simulink library "ECO_TestLibs"  (R2018a)
settings: Solver=ode45  StartTime=0.0  StopTime=10.0  RelTol=1e-3  EnableMultiTasking=on
undefined symbols (not defined in the file or in its folder): h, km
libraries: CoderSF_BSW_Libs x643, $bdroot x217, SF_CanService_Libs x60, simulink x12
(part 2 of 7)

== system ECO_TestLibs/TAF_CANA/Connected ==
  "Read CAN Message " : SF_CanService_Libs/Read CAN Message  typeCAN=Connected  channel=CAN_A  mEn=off  msgInfo=TAF_CAN_new  msgIterm=CAN0x401x  msgItermStore=CAN0x401x  valid=on  stale=on  motoBit=off  setSignalName=off  defineSignalName=on  prefixSignal='rxCANA'  flgValTest=off  flgNoFixed=off  tSample=Task_L10ms  modeCode=Parameterless
  "Read Fixed-Point CAN Message " : SF_CanService_Libs/Read Fixed-Point CAN Message   typeCAN=Connected  channel=CAN_A  mEn=off  msgInfo=TAF_CAN_new  msgIterm=CAN0x401  msgItermStore=CAN0x401  valid=on  stale=on  motoBit=off  setSignalName=on  defineSignalName=on  prefixSignal='rxCANA'  flgValTest=off  flgNoFixed=off  tSample=Task_L10ms  modeCode=Parameterless
  Subsystem : Subsystem
  Subsystem1 : Subsystem
  Write Measurement1 : CoderSF_BSW_Libs/Calibration & Measurement/Write Measurement  variable_name=TAF_CANF_cntCANARx  variable_value=0  variable_type=uint32  numD=1  unitStr=""  descStr=""
      settings: AttributesFormatString=value:%<variable_value> type:%<variable_type>  SourceProductName=EcoCoder Blocks
  Write Measurement2 : CoderSF_BSW_Libs/Calibration & Measurement/Write Measurement  variable_name=TAF_CAN_cntCANARx  variable_value=0  variable_type=uint32  numD=1  unitStr=""  descStr=""
      settings: AttributesFormatString=value:%<variable_value> type:%<variable_type>  SourceProductName=EcoCoder Blocks
  wires:
  "Read CAN Message "/1 -> Subsystem1/Enable
  "Read CAN Message "/2 -> Write Measurement2/1
  "Read CAN Message "/3 -> Subsystem1/1(In1)
  "Read CAN Message "/4 -> Subsystem1/2(In2)
  "Read CAN Message "/5 -> Subsystem1/3(In3)
  "Read CAN Message "/6 -> Subsystem1/4(In4)
  "Read CAN Message "/7 -> Subsystem1/5(In5)
  "Read CAN Message "/8 -> Subsystem1/6(In6)
  "Read CAN Message "/9 -> Subsystem1/7(In7)
  "Read CAN Message "/10 -> Subsystem1/8(In8)
  "Read Fixed-Point CAN Message "/10 -> Subsystem/8(In8)  "rxCANAByte0"
  "Read Fixed-Point CAN Message "/9 -> Subsystem/7(In7)  "rxCANAByte1"
  "Read Fixed-Point CAN Message "/8 -> Subsystem/6(In6)  "rxCANAByte2"
  "Read Fixed-Point CAN Message "/7 -> Subsystem/5(In5)  "rxCANAByte3"
  "Read Fixed-Point CAN Message "/6 -> Subsystem/4(In4)  "rxCANAByte4"
  "Read Fixed-Point CAN Message "/5 -> Subsystem/3(In3)  "rxCANAByte5"
  "Read Fixed-Point CAN Message "/4 -> Subsystem/2(In2)  "rxCANAByte6"
  "Read Fixed-Point CAN Message "/3 -> Subsystem/1(In1)  "rxCANAByte7"
  "Read Fixed-Point CAN Message "/2 -> Write Measurement1/1
  "Read Fixed-Point CAN Message "/1 -> Subsystem/Enable

== system ECO_TestLibs/TAF_CANA/Disconnected ==
  "Read CAN Message " : SF_CanService_Libs/Read CAN Message  typeCAN=Disconnected  channel=CAN_A  mEn=off  msgInfo=TAF_CAN_new  msgIterm=CAN0x402x  msgItermStore=CAN0x402x  valid=on  stale=on  motoBit=off  setSignalName=off  defineSignalName=on  prefixSignal='rxCANA'  flgValTest=off  flgNoFixed=off  tSample=Task_L10ms  modeCode=Parameterless
  "Read Fixed-Point CAN Message " : SF_CanService_Libs/Read Fixed-Point CAN Message   typeCAN=Disconnected  channel=CAN_A  mEn=off  msgInfo=TAF_CAN_new  msgIterm=CAN0x402  msgItermStore=CAN0x402  valid=on  stale=on  motoBit=off  setSignalName=on  defineSignalName=on  prefixSignal='rxCANA2'  flgValTest=off  flgNoFixed=off  tSample=Task_L10ms  modeCode=Parameterless
  Receive CAN Message : CoderSF_BSW_Libs/CAN/Receive CAN Message  channel=CAN_A  txid=hex2dec('402')  extended=off  txlen=8  tasktimeIndex=Task_Inherit
      settings: SourceProductName=EcoCoder Blocks
  Receive CAN Message1 : CoderSF_BSW_Libs/CAN/Receive CAN Message  channel=CAN_A  txid=hex2dec('412')  extended=on  txlen=8  tasktimeIndex=Task_Inherit
      settings: SourceProductName=EcoCoder Blocks
  Subsystem : Subsystem
  Subsystem1 : Subsystem
  Write Measurement1 : CoderSF_BSW_Libs/Calibration & Measurement/Write Measurement  variable_name=TAF_CANF_cntCANARx2  variable_value=0  variable_type=uint32  numD=1  unitStr=""  descStr=""
      settings: AttributesFormatString=value:%<variable_value> type:%<variable_type>  SourceProductName=EcoCoder Blocks
  Write Measurement2 : CoderSF_BSW_Libs/Calibration & Measurement/Write Measurement  variable_name=TAF_CAN_cntCANARx2  variable_value=0  variable_type=uint32  numD=1  unitStr=""  descStr=""
      settings: AttributesFormatString=value:%<variable_value> type:%<variable_type>  SourceProductName=EcoCoder Blocks
  wires:
  "Read Fixed-Point CAN Message "/1 -> Subsystem/Enable
  "Read Fixed-Point CAN Message "/2 -> Write Measurement1/1
  "Read Fixed-Point CAN Message "/3 -> Subsystem/1(In1)  "rxCANA2Byte7"
  "Read Fixed-Point CAN Message "/4 -> Subsystem/2(In2)  "rxCANA2Byte6"
  "Read Fixed-Point CAN Message "/5 -> Subsystem/3(In3)  "rxCANA2Byte5"
  "Read Fixed-Point CAN Message "/6 -> Subsystem/4(In4)  "rxCANA2Byte4"
  "Read Fixed-Point CAN Message "/7 -> Subsystem/5(In5)  "rxCANA2Byte3"
  "Read Fixed-Point CAN Message "/8 -> Subsystem/6(In6)  "rxCANA2Byte2"
  "Read Fixed-Point CAN Message "/9 -> Subsystem/7(In7)  "rxCANA2Byte1"
  "Read Fixed-Point CAN Message "/10 -> Subsystem/8(In8)  "rxCANA2Byte0"
  "Read CAN Message "/10 -> Subsystem1/8(In8)
  "Read CAN Message "/9 -> Subsystem1/7(In7)
  "Read CAN Message "/8 -> Subsystem1/6(In6)
  "Read CAN Message "/7 -> Subsystem1/5(In5)
  "Read CAN Message "/6 -> Subsystem1/4(In4)
  "Read CAN Message "/5 -> Subsystem1/3(In3)
  "Read CAN Message "/4 -> Subsystem1/2(In2)
  "Read CAN Message "/3 -> Subsystem1/1(In1)
  "Read CAN Message "/2 -> Write Measurement2/1
  "Read CAN Message "/1 -> Subsystem1/Enable
  Receive CAN Message/3 -> "Read Fixed-Point CAN Message "/3
  Receive CAN Message/6 -> "Read Fixed-Point CAN Message "/6
  Receive CAN Message/1 -> "Read Fixed-Point CAN Message "/1
  Receive CAN Message/4 -> "Read Fixed-Point CAN Message "/4
  Receive CAN Message/5 -> "Read Fixed-Point CAN Message "/5
  Receive CAN Message/2 -> "Read Fixed-Point CAN Message "/2
  Receive CAN Message1/3 -> "Read CAN Message "/3
  Receive CAN Message1/4 -> "Read CAN Message "/4
  Receive CAN Message1/2 -> "Read CAN Message "/2
  Receive CAN Message1/5 -> "Read CAN Message "/5
  Receive CAN Message1/1 -> "Read CAN Message "/1
  Receive CAN Message1/6 -> "Read CAN Message "/6

== system ECO_TestLibs/TAF_CANA/Enabled Subsystem ==
  In1 : Inport
  Enable : EnablePort
  "Send CAN Message " : SF_CanService_Libs/Send CAN Message   typeCAN=Connected  channel=CAN_A  mEn=off  msgInfo=TAF_CAN_new  msgIterm=CAN0x7ff  msgItermStore=CAN0x7ff  motoBit=off  flgNoFixed=off  tSample=Task_MDef  modeCode=Parameterless
  Send CAN Message 1 : SF_CanService_Libs/Send CAN Message   typeCAN=Connected  channel=CAN_A  mEn=off  msgInfo=TAF_CAN_new  msgIterm=CAN0x1fffffff  msgItermStore=CAN0x1fffffff  motoBit=off  flgNoFixed=off  tSample=Task_MDef  modeCode=Parameterless
  wires:
  In1/1 -> Send CAN Message 1/1, "Send CAN Message "/1

== system ECO_TestLibs/TAF_CANA/Receive CAN Message ==
  Receive CAN Message : CoderSF_BSW_Libs/CAN/Receive CAN Message  channel=CAN_A  txid=hex2dec('100')  extended=off  txlen=8  tasktimeIndex=Task_L1ms
      settings: SourceProductName=EcoCoder Blocks
  Receive CAN Message1 : CoderSF_BSW_Libs/CAN/Receive CAN Message  channel=CAN_A  txid=hex2dec('100')  extended=off  txlen=8  tasktimeIndex=Task_L1ms
      settings: SourceProductName=EcoCoder Blocks
  Receive CAN Message2 : CoderSF_BSW_Libs/CAN/Receive CAN Message  channel=CAN_A  txid=hex2dec('100')  extended=off  txlen=8  tasktimeIndex=Task_L1ms
      settings: SourceProductName=EcoCoder Blocks
  Write Measurement1 : CoderSF_BSW_Libs/Calibration & Measurement/Write Measurement  variable_name=CANAR1_flgAvailable  variable_value=0  variable_type=boolean  numD=1  unitStr=""  descStr=""
      settings: AttributesFormatString=type:%<variable_type> Dimensions:%<numD>  SourceProductName=EcoCoder Blocks
  Write Measurement10 : CoderSF_BSW_Libs/Calibration & Measurement/Write Measurement  variable_name=CANAR2_id  variable_value=0  variable_type=uint32  numD=1  unitStr=""  descStr=""
      settings: AttributesFormatString=type:%<variable_type> Dimensions:%<numD>  SourceProductName=EcoCoder Blocks
  Write Measurement11 : CoderSF_BSW_Libs/Calibration & Measurement/Write Measurement  variable_name=CANAR2_len  variable_value=0  variable_type=uint8  numD=1  unitStr=""  descStr=""
      settings: AttributesFormatString=type:%<variable_type> Dimensions:%<numD>  SourceProductName=EcoCoder Blocks
  Write Measurement12 : CoderSF_BSW_Libs/Calibration & Measurement/Write Measurement  variable_name=CANAR2_data  variable_value=0  variable_type=uint8  numD=8  unitStr=""  descStr=""
      settings: AttributesFormatString=type:%<variable_type> Dimensions:%<numD>  SourceProductName=EcoCoder Blocks
  Write Measurement13 : CoderSF_BSW_Libs/Calibration & Measurement/Write Measurement  variable_name=CANAR3_id  variable_value=0  variable_type=uint32  numD=1  unitStr=""  descStr=""
      settings: AttributesFormatString=type:%<variable_type> Dimensions:%<numD>  SourceProductName=EcoCoder Blocks
  Write Measurement14 : CoderSF_BSW_Libs/Calibration & Measurement/Write Measurement  variable_name=CANAR3_len  variable_value=0  variable_type=uint8  numD=1  unitStr=""  descStr=""
      settings: AttributesFormatString=type:%<variable_type> Dimensions:%<numD>  SourceProductName=EcoCoder Blocks
  Write Measurement15 : CoderSF_BSW_Libs/Calibration & Measurement/Write Measurement  variable_name=CANAR3_data  variable_value=0  variable_type=uint8  numD=8  unitStr=""  descStr=""
      settings: AttributesFormatString=type:%<variable_type> Dimensions:%<numD>  SourceProductName=EcoCoder Blocks
  Write Measurement16 : CoderSF_BSW_Libs/Calibration & Measurement/Write Measurement  variable_name=CANAR3_flgAvailable  variable_value=0  variable_type=boolean  numD=1  unitStr=""  descStr=""
      settings: AttributesFormatString=type:%<variable_type> Dimensions:%<numD>  SourceProductName=EcoCoder Blocks
  Write Measurement17 : CoderSF_BSW_Libs/Calibration & Measurement/Write Measurement  variable_name=CANAR3_flgRemote  variable_value=0  variable_type=boolean  numD=1  unitStr=""  descStr=""
      settings: AttributesFormatString=type:%<variable_type> Dimensions:%<numD>  SourceProductName=EcoCoder Blocks
  Write Measurement18 : CoderSF_BSW_Libs/Calibration & Measurement/Write Measurement  variable_name=CANAR3_flgExtend  variable_value=0  variable_type=boolean  numD=1  unitStr=""  descStr=""
      settings: AttributesFormatString=type:%<variable_type> Dimensions:%<numD>  SourceProductName=EcoCoder Blocks
  Write Measurement19 : CoderSF_BSW_Libs/Calibration & Measurement/Write Measurement  variable_name=CANAR2_flgExtend  variable_value=0  variable_type=boolean  numD=1  unitStr=""  descStr=""
      settings: AttributesFormatString=type:%<variable_type> Dimensions:%<numD>  SourceProductName=EcoCoder Blocks
  Write Measurement3 : CoderSF_BSW_Libs/Calibration & Measurement/Write Measurement  variable_name=CANAR1_flgRemote  variable_value=0  variable_type=boolean  numD=1  unitStr=""  descStr=""
      settings: AttributesFormatString=type:%<variable_type> Dimensions:%<numD>  SourceProductName=EcoCoder Blocks
  Write Measurement4 : CoderSF_BSW_Libs/Calibration & Measurement/Write Measurement  variable_name=CANAR1_flgExtend  variable_value=0  variable_type=boolean  numD=1  unitStr=""  descStr=""
      settings: AttributesFormatString=type:%<variable_type> Dimensions:%<numD>  SourceProductName=EcoCoder Blocks
  Write Measurement5 : CoderSF_BSW_Libs/Calibration & Measurement/Write Measurement  variable_name=CANAR1_id  variable_value=0  variable_type=uint32  numD=1  unitStr=""  descStr=""
      settings: AttributesFormatString=type:%<variable_type> Dimensions:%<numD>  SourceProductName=EcoCoder Blocks
  Write Measurement6 : CoderSF_BSW_Libs/Calibration & Measurement/Write Measurement  variable_name=CANAR1_len  variable_value=0  variable_type=uint8  numD=1  unitStr=""  descStr=""
      settings: AttributesFormatString=type:%<variable_type> Dimensions:%<numD>  SourceProductName=EcoCoder Blocks
  Write Measurement7 : CoderSF_BSW_Libs/Calibration & Measurement/Write Measurement  variable_name=CANAR1_data  variable_value=0  variable_type=uint8  numD=8  unitStr=""  descStr=""
      settings: AttributesFormatString=type:%<variable_type> Dimensions:%<numD>  SourceProductName=EcoCoder Blocks
  Write Measurement8 : CoderSF_BSW_Libs/Calibration & Measurement/Write Measurement  variable_name=CANAR2_flgAvailable  variable_value=0  variable_type=boolean  numD=1  unitStr=""  descStr=""
      settings: AttributesFormatString=type:%<variable_type> Dimensions:%<numD>  SourceProductName=EcoCoder Blocks
  Write Measurement9 : CoderSF_BSW_Libs/Calibration & Measurement/Write Measurement  variable_name=CANAR2_flgRemote  variable_value=0  variable_type=boolean  numD=1  unitStr=""  descStr=""
      settings: AttributesFormatString=type:%<variable_type> Dimensions:%<numD>  SourceProductName=EcoCoder Blocks
  wires:
  Receive CAN Message/1 -> Write Measurement1/1
  Receive CAN Message/2 -> Write Measurement3/1
  Receive CAN Message/3 -> Write Measurement4/1
  Receive CAN Message/4 -> Write Measurement5/1
  Receive CAN Message/5 -> Write Measurement6/1
  Receive CAN Message/6 -> Write Measurement7/1
  Receive CAN Message1/6 -> Write Measurement12/1
  Receive CAN Message1/4 -> Write Measurement10/1
  Receive CAN Message1/1 -> Write Measurement8/1
  Receive CAN Message1/5 -> Write Measurement11/1
  Receive CAN Message1/2 -> Write Measurement9/1
  Receive CAN Message1/3 -> Write Measurement19/1
  Receive CAN Message2/6 -> Write Measurement15/1
  Receive CAN Message2/4 -> Write Measurement13/1
  Receive CAN Message2/1 -> Write Measurement16/1
  Receive CAN Message2/5 -> Write Measurement14/1
  Receive CAN Message2/2 -> Write Measurement17/1
  Receive CAN Message2/3 -> Write Measurement18/1

== system ECO_TestLibs/TAF_CANA/Subsystem ==
  In1 : Inport
  Logical Operator : Logic  AllPortsSameDT=off  OutDataTypeStr=boolean
  Read Calibration : CoderSF_BSW_Libs/Calibration & Measurement/Read Calibration  variable_name=TAF_CANA_flgEnRxResp_val  variable_value=1  variable_type=boolean  variable_min=[]  variable_max=[]  unitStr=""  descStr=""
      settings: AttributesFormatString=value:%<variable_value> type:%<variable_type> max:%<variable_max> Min:%<variable_min>  SourceProductName=EcoCoder Blocks
  Out1 : Outport
  wires:
  Logical Operator/1 -> Out1/1
  Read Calibration/1 -> Logical Operator/1
  In1/1 -> Logical Operator/2

== system ECO_TestLibs/TAF_CANB/Connected ==
  Read CAN Message 1 : SF_CanService_Libs/Read CAN Message  typeCAN=Connected  channel=CAN_B  mEn=off  msgInfo=TAF_CAN_new  msgIterm=CAN0x403x  msgItermStore=CAN0x403x  valid=on  stale=on  motoBit=off  setSignalName=off  defineSignalName=on  prefixSignal='rxCANB'  flgValTest=off  flgNoFixed=off  tSample=Task_L10ms  modeCode=Parameterless
  Read Fixed-Point CAN Message 1 : SF_CanService_Libs/Read Fixed-Point CAN Message   typeCAN=Connected  channel=CAN_B  mEn=off  msgInfo=TAF_CAN_new  msgIterm=CAN0x403  msgItermStore=CAN0x403  valid=on  stale=on  motoBit=off  setSignalName=on  defineSignalName=on  prefixSignal='rxCANB'  flgValTest=off  flgNoFixed=off  tSample=Task_L10ms  modeCode=Parameterless
  Subsystem1 : Subsystem
  Subsystem5 : Subsystem
  Write Measurement5 : CoderSF_BSW_Libs/Calibration & Measurement/Write Measurement  variable_name=TAF_CAN_cntCANBRx  variable_value=0  variable_type=uint32  numD=1  unitStr=""  descStr=""
      settings: AttributesFormatString=value:%<variable_value> type:%<variable_type>  SourceProductName=EcoCoder Blocks
  Write Measurement6 : CoderSF_BSW_Libs/Calibration & Measurement/Write Measurement  variable_name=TAF_CANF_cntCANBRx  variable_value=0  variable_type=uint32  numD=1  unitStr=""  descStr=""
      settings: AttributesFormatString=value:%<variable_value> type:%<variable_type>  SourceProductName=EcoCoder Blocks
  wires:
  Read Fixed-Point CAN Message 1/4 -> Subsystem1/2(In2)  "rxCANBByte6"
  Read CAN Message 1/1 -> Subsystem5/Enable
  Read CAN Message 1/2 -> Write Measurement5/1
  Read CAN Message 1/3 -> Subsystem5/1(In1)
  Read CAN Message 1/4 -> Subsystem5/2(In2)
  Read CAN Message 1/5 -> Subsystem5/3(In3)
  Read CAN Message 1/6 -> Subsystem5/4(In4)
  Read CAN Message 1/7 -> Subsystem5/5(In5)
  Read CAN Message 1/8 -> Subsystem5/6(In6)
  Read CAN Message 1/9 -> Subsystem5/7(In7)
  Read CAN Message 1/10 -> Subsystem5/8(In8)
  Read Fixed-Point CAN Message 1/10 -> Subsystem1/8(In8)  "rxCANBByte0"
  Read Fixed-Point CAN Message 1/9 -> Subsystem1/7(In7)  "rxCANBByte1"
  Read Fixed-Point CAN Message 1/8 -> Subsystem1/6(In6)  "rxCANBByte2"
  Read Fixed-Point CAN Message 1/7 -> Subsystem1/5(In5)  "rxCANBByte3"
  Read Fixed-Point CAN Message 1/6 -> Subsystem1/4(In4)  "rxCANBByte4"
  Read Fixed-Point CAN Message 1/5 -> Subsystem1/3(In3)  "rxCANBByte5"
  Read Fixed-Point CAN Message 1/3 -> Subsystem1/1(In1)  "rxCANBByte7"
  Read Fixed-Point CAN Message 1/2 -> Write Measurement6/1
  Read Fixed-Point CAN Message 1/1 -> Subsystem1/Enable

== system ECO_TestLibs/TAF_CANB/Disconnected ==
  Read CAN Message 1 : SF_CanService_Libs/Read CAN Message  typeCAN=Disconnected  channel=CAN_B  mEn=off  msgInfo=TAF_CAN_new  msgIterm=CAN0x404x  msgItermStore=CAN0x404x  valid=on  stale=on  motoBit=off  setSignalName=off  defineSignalName=on  prefixSignal='rxCANB'  flgValTest=off  flgNoFixed=off  tSample=Task_L10ms  modeCode=Parameterless
  Read Fixed-Point CAN Message 1 : SF_CanService_Libs/Read Fixed-Point CAN Message   typeCAN=Disconnected  channel=CAN_B  mEn=off  msgInfo=TAF_CAN_new  msgIterm=CAN0x404  msgItermStore=CAN0x404  valid=on  stale=on  motoBit=off  setSignalName=on  defineSignalName=on  prefixSignal='rxCANB2'  flgValTest=off  flgNoFixed=off  tSample=Task_L10ms  modeCode=Parameterless
  Receive CAN Message : CoderSF_BSW_Libs/CAN/Receive CAN Message  channel=CAN_B  txid=hex2dec('404')  extended=off  txlen=8  tasktimeIndex=Task_Inherit
      settings: SourceProductName=EcoCoder Blocks
  Receive CAN Message1 : CoderSF_BSW_Libs/CAN/Receive CAN Message  channel=CAN_B  txid=hex2dec('414')  extended=on  txlen=8  tasktimeIndex=Task_Inherit
      settings: SourceProductName=EcoCoder Blocks
  Subsystem1 : Subsystem
  Subsystem5 : Subsystem
  Write Measurement5 : CoderSF_BSW_Libs/Calibration & Measurement/Write Measurement  variable_name=TAF_CAN_cntCANBRx2  variable_value=0  variable_type=uint32  numD=1  unitStr=""  descStr=""
      settings: AttributesFormatString=value:%<variable_value> type:%<variable_type>  SourceProductName=EcoCoder Blocks
  Write Measurement6 : CoderSF_BSW_Libs/Calibration & Measurement/Write Measurement  variable_name=TAF_CANF_cntCANBRx2  variable_value=0  variable_type=uint32  numD=1  unitStr=""  descStr=""
      settings: AttributesFormatString=value:%<variable_value> type:%<variable_type>  SourceProductName=EcoCoder Blocks
  wires:
  Read Fixed-Point CAN Message 1/1 -> Subsystem1/Enable
  Read Fixed-Point CAN Message 1/2 -> Write Measurement6/1
  Read Fixed-Point CAN Message 1/3 -> Subsystem1/1(In1)  "rxCANB2Byte7"
  Read Fixed-Point CAN Message 1/5 -> Subsystem1/3(In3)  "rxCANB2Byte5"
  Read Fixed-Point CAN Message 1/6 -> Subsystem1/4(In4)  "rxCANB2Byte4"
  Read Fixed-Point CAN Message 1/7 -> Subsystem1/5(In5)  "rxCANB2Byte3"
  Read Fixed-Point CAN Message 1/8 -> Subsystem1/6(In6)  "rxCANB2Byte2"
  Read Fixed-Point CAN Message 1/9 -> Subsystem1/7(In7)  "rxCANB2Byte1"
  Read Fixed-Point CAN Message 1/10 -> Subsystem1/8(In8)  "rxCANB2Byte0"
  Read CAN Message 1/10 -> Subsystem5/8(In8)
  Read CAN Message 1/9 -> Subsystem5/7(In7)
  Read CAN Message 1/8 -> Subsystem5/6(In6)
  Read CAN Message 1/7 -> Subsystem5/5(In5)
  Read CAN Message 1/6 -> Subsystem5/4(In4)
  Read CAN Message 1/5 -> Subsystem5/3(In3)
  Read CAN Message 1/4 -> Subsystem5/2(In2)
  Read CAN Message 1/3 -> Subsystem5/1(In1)
  Read CAN Message 1/2 -> Write Measurement5/1
  Read CAN Message 1/1 -> Subsystem5/Enable
  Read Fixed-Point CAN Message 1/4 -> Subsystem1/2(In2)  "rxCANB2Byte6"
  Receive CAN Message/5 -> Read Fixed-Point CAN Message 1/5
  Receive CAN Message/6 -> Read Fixed-Point CAN Message 1/6
  Receive CAN Message/3 -> Read Fixed-Point CAN Message 1/3
  Receive CAN Message/2 -> Read Fixed-Point CAN Message 1/2
  Receive CAN Message/4 -> Read Fixed-Point CAN Message 1/4
  Receive CAN Message/1 -> Read Fixed-Point CAN Message 1/1
  Receive CAN Message1/3 -> Read CAN Message 1/3
  Receive CAN Message1/5 -> Read CAN Message 1/5
  Receive CAN Message1/2 -> Read CAN Message 1/2
  Receive CAN Message1/1 -> Read CAN Message 1/1
  Receive CAN Message1/6 -> Read CAN Message 1/6
  Receive CAN Message1/4 -> Read CAN Message 1/4

== system ECO_TestLibs/TAF_CANB/Enabled Subsystem ==
  In1 : Inport
  Enable : EnablePort
  "Send CAN Message " : SF_CanService_Libs/Send CAN Message   typeCAN=Connected  channel=CAN_B  mEn=off  msgInfo=TAF_CAN_new  msgIterm=CAN0x7fe  msgItermStore=CAN0x7fe  motoBit=off  flgNoFixed=off  tSample=Task_MDef  modeCode=Parameterless
  Send CAN Message 1 : SF_CanService_Libs/Send CAN Message   typeCAN=Connected  channel=CAN_B  mEn=off  msgInfo=TAF_CAN_new  msgIterm=CAN0x1ffffffe  msgItermStore=CAN0x1ffffffe  motoBit=off  flgNoFixed=off  tSample=Task_MDef  modeCode=Parameterless
  wires:
  In1/1 -> Send CAN Message 1/1, "Send CAN Message "/1

== system ECO_TestLibs/TAF_CANB/Receive CAN Message ==
  Receive CAN Message : CoderSF_BSW_Libs/CAN/Receive CAN Message  channel=CAN_B  txid=hex2dec('100')  extended=off  txlen=8  tasktimeIndex=Task_L1ms
      settings: SourceProductName=EcoCoder Blocks
  Receive CAN Message1 : CoderSF_BSW_Libs/CAN/Receive CAN Message  channel=CAN_B  txid=hex2dec('100')  extended=off  txlen=8  tasktimeIndex=Task_L1ms
      settings: SourceProductName=EcoCoder Blocks
  Receive CAN Message2 : CoderSF_BSW_Libs/CAN/Receive CAN Message  channel=CAN_B  txid=hex2dec('100')  extended=off  txlen=8  tasktimeIndex=Task_L1ms
      settings: SourceProductName=EcoCoder Blocks
  Write Measurement1 : CoderSF_BSW_Libs/Calibration & Measurement/Write Measurement  variable_name=CANBR1_flgAvailable  variable_value=0  variable_type=boolean  numD=1  unitStr=""  descStr=""
      settings: AttributesFormatString=type:%<variable_type> Dimensions:%<numD>  SourceProductName=EcoCoder Blocks
  Write Measurement10 : CoderSF_BSW_Libs/Calibration & Measurement/Write Measurement  variable_name=CANBR2_id  variable_value=0  variable_type=uint32  numD=1  unitStr=""  descStr=""
      settings: AttributesFormatString=type:%<variable_type> Dimensions:%<numD>  SourceProductName=EcoCoder Blocks
  Write Measurement11 : CoderSF_BSW_Libs/Calibration & Measurement/Write Measurement  variable_name=CANBR2_len  variable_value=0  variable_type=uint8  numD=1  unitStr=""  descStr=""
      settings: AttributesFormatString=type:%<variable_type> Dimensions:%<numD>  SourceProductName=EcoCoder Blocks
  Write Measurement12 : CoderSF_BSW_Libs/Calibration & Measurement/Write Measurement  variable_name=CANBR2_data  variable_value=0  variable_type=uint8  numD=8  unitStr=""  descStr=""
      settings: AttributesFormatString=type:%<variable_type> Dimensions:%<numD>  SourceProductName=EcoCoder Blocks
  Write Measurement13 : CoderSF_BSW_Libs/Calibration & Measurement/Write Measurement  variable_name=CANBR3_id  variable_value=0  variable_type=uint32  numD=1  unitStr=""  descStr=""
      settings: AttributesFormatString=type:%<variable_type> Dimensions:%<numD>  SourceProductName=EcoCoder Blocks
  Write Measurement14 : CoderSF_BSW_Libs/Calibration & Measurement/Write Measurement  variable_name=CANBR3_len  variable_value=0  variable_type=uint8  numD=1  unitStr=""  descStr=""
      settings: AttributesFormatString=type:%<variable_type> Dimensions:%<numD>  SourceProductName=EcoCoder Blocks
  Write Measurement15 : CoderSF_BSW_Libs/Calibration & Measurement/Write Measurement  variable_name=CANBR3_data  variable_value=0  variable_type=uint8  numD=8  unitStr=""  descStr=""
      settings: AttributesFormatString=type:%<variable_type> Dimensions:%<numD>  SourceProductName=EcoCoder Blocks
  Write Measurement16 : CoderSF_BSW_Libs/Calibration & Measurement/Write Measurement  variable_name=CANBR3_flgAvailable  variable_value=0  variable_type=boolean  numD=1  unitStr=""  descStr=""
      settings: AttributesFormatString=type:%<variable_type> Dimensions:%<numD>  SourceProductName=EcoCoder Blocks
  Write Measurement17 : CoderSF_BSW_Libs/Calibration & Measurement/Write Measurement  variable_name=CANBR3_flgRemote  variable_value=0  variable_type=boolean  numD=1  unitStr=""  descStr=""
      settings: AttributesFormatString=type:%<variable_type> Dimensions:%<numD>  SourceProductName=EcoCoder Blocks
  Write Measurement18 : CoderSF_BSW_Libs/Calibration & Measurement/Write Measurement  variable_name=CANBR3_flgExtend  variable_value=0  variable_type=boolean  numD=1  unitStr=""  descStr=""
      settings: AttributesFormatString=type:%<variable_type> Dimensions:%<numD>  SourceProductName=EcoCoder Blocks
  Write Measurement19 : CoderSF_BSW_Libs/Calibration & Measurement/Write Measurement  variable_name=CANBR2_flgExtend  variable_value=0  variable_type=boolean  numD=1  unitStr=""  descStr=""
      settings: AttributesFormatString=type:%<variable_type> Dimensions:%<numD>  SourceProductName=EcoCoder Blocks
  Write Measurement3 : CoderSF_BSW_Libs/Calibration & Measurement/Write Measurement  variable_name=CANBR1_flgRemote  variable_value=0  variable_type=boolean  numD=1  unitStr=""  descStr=""
      settings: AttributesFormatString=type:%<variable_type> Dimensions:%<numD>  SourceProductName=EcoCoder Blocks
  Write Measurement4 : CoderSF_BSW_Libs/Calibration & Measurement/Write Measurement  variable_name=CANBR1_flgExtend  variable_value=0  variable_type=boolean  numD=1  unitStr=""  descStr=""
      settings: AttributesFormatString=type:%<variable_type> Dimensions:%<numD>  SourceProductName=EcoCoder Blocks
  Write Measurement5 : CoderSF_BSW_Libs/Calibration & Measurement/Write Measurement  variable_name=CANBR1_id  variable_value=0  variable_type=uint32  numD=1  unitStr=""  descStr=""
      settings: AttributesFormatString=type:%<variable_type> Dimensions:%<numD>  SourceProductName=EcoCoder Blocks
  Write Measurement6 : CoderSF_BSW_Libs/Calibration & Measurement/Write Measurement  variable_name=CANBR1_len  variable_value=0  variable_type=uint8  numD=1  unitStr=""  descStr=""
      settings: AttributesFormatString=type:%<variable_type> Dimensions:%<numD>  SourceProductName=EcoCoder Blocks
  Write Measurement7 : CoderSF_BSW_Libs/Calibration & Measurement/Write Measurement  variable_name=CANBR1_data  variable_value=0  variable_type=uint8  numD=8  unitStr=""  descStr=""
      settings: AttributesFormatString=type:%<variable_type> Dimensions:%<numD>  SourceProductName=EcoCoder Blocks
  Write Measurement8 : CoderSF_BSW_Libs/Calibration & Measurement/Write Measurement  variable_name=CANBR2_flgAvailable  variable_value=0  variable_type=boolean  numD=1  unitStr=""  descStr=""
      settings: AttributesFormatString=type:%<variable_type> Dimensions:%<numD>  SourceProductName=EcoCoder Blocks
  Write Measurement9 : CoderSF_BSW_Libs/Calibration & Measurement/Write Measurement  variable_name=CANBR2_flgRemote  variable_value=0  variable_type=boolean  numD=1  unitStr=""  descStr=""
      settings: AttributesFormatString=type:%<variable_type> Dimensions:%<numD>  SourceProductName=EcoCoder Blocks
  wires:
  Receive CAN Message/1 -> Write Measurement1/1
  Receive CAN Message/2 -> Write Measurement3/1
  Receive CAN Message/3 -> Write Measurement4/1
  Receive CAN Message/4 -> Write Measurement5/1
  Receive CAN Message/5 -> Write Measurement6/1
  Receive CAN Message/6 -> Write Measurement7/1
  Receive CAN Message1/6 -> Write Measurement12/1
  Receive CAN Message1/4 -> Write Measurement10/1
  Receive CAN Message1/1 -> Write Measurement8/1
  Receive CAN Message1/5 -> Write Measurement11/1
  Receive CAN Message1/2 -> Write Measurement9/1
  Receive CAN Message1/3 -> Write Measurement19/1
  Receive CAN Message2/6 -> Write Measurement15/1
  Receive CAN Message2/4 -> Write Measurement13/1
  Receive CAN Message2/1 -> Write Measurement16/1
  Receive CAN Message2/5 -> Write Measurement14/1
  Receive CAN Message2/2 -> Write Measurement17/1
  Receive CAN Message2/3 -> Write Measurement18/1

== system ECO_TestLibs/TAF_CANB/Subsystem ==
  In1 : Inport
  Logical Operator : Logic  AllPortsSameDT=off  OutDataTypeStr=boolean
  Read Calibration : CoderSF_BSW_Libs/Calibration & Measurement/Read Calibration  variable_name=TAF_CANB_flgEnRxResp_val  variable_value=1  variable_type=boolean  variable_min=[]  variable_max=[]  unitStr=""  descStr=""
      settings: AttributesFormatString=value:%<variable_value> type:%<variable_type> max:%<variable_max> Min:%<variable_min>  SourceProductName=EcoCoder Blocks
  Out1 : Outport
  wires:
  Logical Operator/1 -> Out1/1
  Read Calibration/1 -> Logical Operator/1
  In1/1 -> Logical Operator/2

== system ECO_TestLibs/TAF_CANC/Connected ==
  Read CAN Message 2 : SF_CanService_Libs/Read CAN Message  typeCAN=Connected  channel=CAN_C  mEn=off  msgInfo=TAF_CAN_new  msgIterm=CAN0x405x  msgItermStore=CAN0x405x  valid=on  stale=on  motoBit=off  setSignalName=off  defineSignalName=on  prefixSignal='rxCANC'  flgValTest=off  flgNoFixed=off  tSample=Task_L10ms  modeCode=Parameterless
  Read Fixed-Point CAN Message 2 : SF_CanService_Libs/Read Fixed-Point CAN Message   typeCAN=Connected  channel=CAN_C  mEn=off  msgInfo=TAF_CAN_new  msgIterm=CAN0x405  msgItermStore=CAN0x405  valid=on  stale=on  motoBit=off  setSignalName=on  defineSignalName=on  prefixSignal='rxCANC'  flgValTest=off  flgNoFixed=off  tSample=Task_L10ms  modeCode=Parameterless
  Subsystem2 : Subsystem
  Subsystem6 : Subsystem
  Write Measurement10 : CoderSF_BSW_Libs/Calibration & Measurement/Write Measurement  variable_name=TAF_CAN_cntCANCRx  variable_value=0  variable_type=uint32  numD=1  unitStr=""  descStr=""
      settings: AttributesFormatString=value:%<variable_value> type:%<variable_type>  SourceProductName=EcoCoder Blocks
  Write Measurement7 : CoderSF_BSW_Libs/Calibration & Measurement/Write Measurement  variable_name=TAF_CANF_cntCANCRx  variable_value=0  variable_type=uint32  numD=1  unitStr=""  descStr=""
      settings: AttributesFormatString=value:%<variable_value> type:%<variable_type>  SourceProductName=EcoCoder Blocks
  wires:
  Read Fixed-Point CAN Message 2/1 -> Subsystem2/Enable
  Read Fixed-Point CAN Message 2/2 -> Write Measurement7/1
  Read Fixed-Point CAN Message 2/3 -> Subsystem2/1(In1)  "rxCANCByte7"
  Read Fixed-Point CAN Message 2/4 -> Subsystem2/2(In2)  "rxCANCByte6"
  Read Fixed-Point CAN Message 2/5 -> Subsystem2/3(In3)  "rxCANCByte5"
  Read Fixed-Point CAN Message 2/6 -> Subsystem2/4(In4)  "rxCANCByte4"
  Read Fixed-Point CAN Message 2/7 -> Subsystem2/5(In5)  "rxCANCByte3"
  Read Fixed-Point CAN Message 2/8 -> Subsystem2/6(In6)  "rxCANCByte2"
  Read Fixed-Point CAN Message 2/9 -> Subsystem2/7(In7)  "rxCANCByte1"
  Read Fixed-Point CAN Message 2/10 -> Subsystem2/8(In8)  "rxCANCByte0"
  Read CAN Message 2/10 -> Subsystem6/8(In8)
  Read CAN Message 2/9 -> Subsystem6/7(In7)
  Read CAN Message 2/8 -> Subsystem6/6(In6)
  Read CAN Message 2/7 -> Subsystem6/5(In5)
  Read CAN Message 2/6 -> Subsystem6/4(In4)
  Read CAN Message 2/5 -> Subsystem6/3(In3)
  Read CAN Message 2/4 -> Subsystem6/2(In2)
  Read CAN Message 2/3 -> Subsystem6/1(In1)
  Read CAN Message 2/2 -> Write Measurement10/1
  Read CAN Message 2/1 -> Subsystem6/Enable

== system ECO_TestLibs/TAF_CANC/Disconnected ==
  Read CAN Message 2 : SF_CanService_Libs/Read CAN Message  typeCAN=Disconnected  channel=CAN_C  mEn=off  msgInfo=TAF_CAN_new  msgIterm=CAN0x406x  msgItermStore=CAN0x406x  valid=on  stale=on  motoBit=off  setSignalName=off  defineSignalName=on  prefixSignal='rxCANC'  flgValTest=off  flgNoFixed=off  tSample=Task_L10ms  modeCode=Parameterless
  Read Fixed-Point CAN Message 2 : SF_CanService_Libs/Read Fixed-Point CAN Message   typeCAN=Disconnected  channel=CAN_C  mEn=off  msgInfo=TAF_CAN_new  msgIterm=CAN0x406  msgItermStore=CAN0x406  valid=on  stale=on  motoBit=off  setSignalName=on  defineSignalName=on  prefixSignal='rxCANC2'  flgValTest=off  flgNoFixed=off  tSample=Task_L10ms  modeCode=Parameterless
  Receive CAN Message : CoderSF_BSW_Libs/CAN/Receive CAN Message  channel=CAN_C  txid=hex2dec('406')  extended=off  txlen=8  tasktimeIndex=Task_Inherit
      settings: SourceProductName=EcoCoder Blocks
  Receive CAN Message1 : CoderSF_BSW_Libs/CAN/Receive CAN Message  channel=CAN_C  txid=hex2dec('416')  extended=on  txlen=8  tasktimeIndex=Task_Inherit
      settings: SourceProductName=EcoCoder Blocks
  Subsystem2 : Subsystem
  Subsystem6 : Subsystem
  Write Measurement10 : CoderSF_BSW_Libs/Calibration & Measurement/Write Measurement  variable_name=TAF_CAN_cntCANCRx2  variable_value=0  variable_type=uint32  numD=1  unitStr=""  descStr=""
      settings: AttributesFormatString=value:%<variable_value> type:%<variable_type>  SourceProductName=EcoCoder Blocks
  Write Measurement7 : CoderSF_BSW_Libs/Calibration & Measurement/Write Measurement  variable_name=TAF_CANF_cntCANCRx2  variable_value=0  variable_type=uint32  numD=1  unitStr=""  descStr=""
      settings: AttributesFormatString=value:%<variable_value> type:%<variable_type>  SourceProductName=EcoCoder Blocks
  wires:
  Read CAN Message 2/1 -> Subsystem6/Enable
  Read CAN Message 2/2 -> Write Measurement10/1
  Read CAN Message 2/3 -> Subsystem6/1(In1)
  Read CAN Message 2/4 -> Subsystem6/2(In2)
  Read CAN Message 2/5 -> Subsystem6/3(In3)
  Read CAN Message 2/6 -> Subsystem6/4(In4)
  Read CAN Message 2/7 -> Subsystem6/5(In5)
  Read CAN Message 2/8 -> Subsystem6/6(In6)
  Read CAN Message 2/9 -> Subsystem6/7(In7)
  Read CAN Message 2/10 -> Subsystem6/8(In8)
  Read Fixed-Point CAN Message 2/10 -> Subsystem2/8(In8)  "rxCANC2Byte0"
  Read Fixed-Point CAN Message 2/9 -> Subsystem2/7(In7)  "rxCANC2Byte1"
  Read Fixed-Point CAN Message 2/8 -> Subsystem2/6(In6)  "rxCANC2Byte2"
  Read Fixed-Point CAN Message 2/7 -> Subsystem2/5(In5)  "rxCANC2Byte3"
  Read Fixed-Point CAN Message 2/6 -> Subsystem2/4(In4)  "rxCANC2Byte4"
  Read Fixed-Point CAN Message 2/5 -> Subsystem2/3(In3)  "rxCANC2Byte5"
  Read Fixed-Point CAN Message 2/4 -> Subsystem2/2(In2)  "rxCANC2Byte6"
  Read Fixed-Point CAN Message 2/3 -> Subsystem2/1(In1)  "rxCANC2Byte7"
  Read Fixed-Point CAN Message 2/2 -> Write Measurement7/1
  Read Fixed-Point CAN Message 2/1 -> Subsystem2/Enable
  Receive CAN Message/1 -> Read Fixed-Point CAN Message 2/1
  Receive CAN Message/6 -> Read Fixed-Point CAN Message 2/6
  Receive CAN Message/2 -> Read Fixed-Point CAN Message 2/2
  Receive CAN Message/5 -> Read Fixed-Point CAN Message 2/5
  Receive CAN Message/4 -> Read Fixed-Point CAN Message 2/4
  Receive CAN Message/3 -> Read Fixed-Point CAN Message 2/3
  Receive CAN Message1/1 -> Read CAN Message 2/1
  Receive CAN Message1/4 -> Read CAN Message 2/4
  Receive CAN Message1/5 -> Read CAN Message 2/5
  Receive CAN Message1/6 -> Read CAN Message 2/6
  Receive CAN Message1/3 -> Read CAN Message 2/3
  Receive CAN Message1/2 -> Read CAN Message 2/2

== system ECO_TestLibs/TAF_CANC/Enabled Subsystem ==
  In1 : Inport
  Enable : EnablePort
  "Send CAN Message " : SF_CanService_Libs/Send CAN Message   typeCAN=Connected  channel=CAN_C  mEn=off  msgInfo=TAF_CAN_new  msgIterm=CAN0x7fd  msgItermStore=CAN0x7fd  motoBit=off  flgNoFixed=off  tSample=Task_MDef  modeCode=Parameterless
  Send CAN Message 1 : SF_CanService_Libs/Send CAN Message   typeCAN=Connected  channel=CAN_C  mEn=off  msgInfo=TAF_CAN_new  msgIterm=CAN0x1ffffffd  msgItermStore=CAN0x1ffffffd  motoBit=off  flgNoFixed=off  tSample=Task_MDef  modeCode=Parameterless
  wires:
  In1/1 -> Send CAN Message 1/1, "Send CAN Message "/1

== system ECO_TestLibs/TAF_CANC/Receive CAN Message ==
  Receive CAN Message : CoderSF_BSW_Libs/CAN/Receive CAN Message  channel=CAN_C  txid=hex2dec('100')  extended=off  txlen=8  tasktimeIndex=Task_L1ms
      settings: SourceProductName=EcoCoder Blocks
  Receive CAN Message1 : CoderSF_BSW_Libs/CAN/Receive CAN Message  channel=CAN_C  txid=hex2dec('100')  extended=off  txlen=8  tasktimeIndex=Task_L1ms
      settings: SourceProductName=EcoCoder Blocks
  Receive CAN Message2 : CoderSF_BSW_Libs/CAN/Receive CAN Message  channel=CAN_C  txid=hex2dec('100')  extended=off  txlen=8  tasktimeIndex=Task_L1ms
      settings: SourceProductName=EcoCoder Blocks
  Write Measurement1 : CoderSF_BSW_Libs/Calibration & Measurement/Write Measurement  variable_name=CANCR1_flgAvailable  variable_value=0  variable_type=boolean  numD=1  unitStr=""  descStr=""
      settings: AttributesFormatString=type:%<variable_type> Dimensions:%<numD>  SourceProductName=EcoCoder Blocks
  Write Measurement10 : CoderSF_BSW_Libs/Calibration & Measurement/Write Measurement  variable_name=CANCR2_id  variable_value=0  variable_type=uint32  numD=1  unitStr=""  descStr=""
      settings: AttributesFormatString=type:%<variable_type> Dimensions:%<numD>  SourceProductName=EcoCoder Blocks
  Write Measurement11 : CoderSF_BSW_Libs/Calibration & Measurement/Write Measurement  variable_name=CANCR2_len  variable_value=0  variable_type=uint8  numD=1  unitStr=""  descStr=""
      settings: AttributesFormatString=type:%<variable_type> Dimensions:%<numD>  SourceProductName=EcoCoder Blocks
  Write Measurement12 : CoderSF_BSW_Libs/Calibration & Measurement/Write Measurement  variable_name=CANCR2_data  variable_value=0  variable_type=uint8  numD=8  unitStr=""  descStr=""
      settings: AttributesFormatString=type:%<variable_type> Dimensions:%<numD>  SourceProductName=EcoCoder Blocks
  Write Measurement13 : CoderSF_BSW_Libs/Calibration & Measurement/Write Measurement  variable_name=CANCR3_id  variable_value=0  variable_type=uint32  numD=1  unitStr=""  descStr=""
      settings: AttributesFormatString=type:%<variable_type> Dimensions:%<numD>  SourceProductName=EcoCoder Blocks
  Write Measurement14 : CoderSF_BSW_Libs/Calibration & Measurement/Write Measurement  variable_name=CANCR3_len  variable_value=0  variable_type=uint8  numD=1  unitStr=""  descStr=""
      settings: AttributesFormatString=type:%<variable_type> Dimensions:%<numD>  SourceProductName=EcoCoder Blocks
  Write Measurement15 : CoderSF_BSW_Libs/Calibration & Measurement/Write Measurement  variable_name=CANCR3_data  variable_value=0  variable_type=uint8  numD=8  unitStr=""  descStr=""
      settings: AttributesFormatString=type:%<variable_type> Dimensions:%<numD>  SourceProductName=EcoCoder Blocks
  Write Measurement16 : CoderSF_BSW_Libs/Calibration & Measurement/Write Measurement  variable_name=CANCR3_flgAvailable  variable_value=0  variable_type=boolean  numD=1  unitStr=""  descStr=""
      settings: AttributesFormatString=type:%<variable_type> Dimensions:%<numD>  SourceProductName=EcoCoder Blocks
  Write Measurement17 : CoderSF_BSW_Libs/Calibration & Measurement/Write Measurement  variable_name=CANCR3_flgRemote  variable_value=0  variable_type=boolean  numD=1  unitStr=""  descStr=""
      settings: AttributesFormatString=type:%<variable_type> Dimensions:%<numD>  SourceProductName=EcoCoder Blocks
  Write Measurement18 : CoderSF_BSW_Libs/Calibration & Measurement/Write Measurement  variable_name=CANCR3_flgExtend  variable_value=0  variable_type=boolean  numD=1  unitStr=""  descStr=""
      settings: AttributesFormatString=type:%<variable_type> Dimensions:%<numD>  SourceProductName=EcoCoder Blocks
  Write Measurement19 : CoderSF_BSW_Libs/Calibration & Measurement/Write Measurement  variable_name=CANCR2_flgExtend  variable_value=0  variable_type=boolean  numD=1  unitStr=""  descStr=""
      settings: AttributesFormatString=type:%<variable_type> Dimensions:%<numD>  SourceProductName=EcoCoder Blocks
  Write Measurement3 : CoderSF_BSW_Libs/Calibration & Measurement/Write Measurement  variable_name=CANCR1_flgRemote  variable_value=0  variable_type=boolean  numD=1  unitStr=""  descStr=""
      settings: AttributesFormatString=type:%<variable_type> Dimensions:%<numD>  SourceProductName=EcoCoder Blocks
  Write Measurement4 : CoderSF_BSW_Libs/Calibration & Measurement/Write Measurement  variable_name=CANCR1_flgExtend  variable_value=0  variable_type=boolean  numD=1  unitStr=""  descStr=""
      settings: AttributesFormatString=type:%<variable_type> Dimensions:%<numD>  SourceProductName=EcoCoder Blocks
  Write Measurement5 : CoderSF_BSW_Libs/Calibration & Measurement/Write Measurement  variable_name=CANCR1_id  variable_value=0  variable_type=uint32  numD=1  unitStr=""  descStr=""
      settings: AttributesFormatString=type:%<variable_type> Dimensions:%<numD>  SourceProductName=EcoCoder Blocks
  Write Measurement6 : CoderSF_BSW_Libs/Calibration & Measurement/Write Measurement  variable_name=CANCR1_len  variable_value=0  variable_type=uint8  numD=1  unitStr=""  descStr=""
      settings: AttributesFormatString=type:%<variable_type> Dimensions:%<numD>  SourceProductName=EcoCoder Blocks
  Write Measurement7 : CoderSF_BSW_Libs/Calibration & Measurement/Write Measurement  variable_name=CANCR1_data  variable_value=0  variable_type=uint8  numD=8  unitStr=""  descStr=""
      settings: AttributesFormatString=type:%<variable_type> Dimensions:%<numD>  SourceProductName=EcoCoder Blocks
  Write Measurement8 : CoderSF_BSW_Libs/Calibration & Measurement/Write Measurement  variable_name=CANCR2_flgAvailable  variable_value=0  variable_type=boolean  numD=1  unitStr=""  descStr=""
      settings: AttributesFormatString=type:%<variable_type> Dimensions:%<numD>  SourceProductName=EcoCoder Blocks
  Write Measurement9 : CoderSF_BSW_Libs/Calibration & Measurement/Write Measurement  variable_name=CANCR2_flgRemote  variable_value=0  variable_type=boolean  numD=1  unitStr=""  descStr=""
      settings: AttributesFormatString=type:%<variable_type> Dimensions:%<numD>  SourceProductName=EcoCoder Blocks
  wires:
  Receive CAN Message/1 -> Write Measurement1/1
  Receive CAN Message/2 -> Write Measurement3/1
  Receive CAN Message/3 -> Write Measurement4/1
  Receive CAN Message/4 -> Write Measurement5/1
  Receive CAN Message/5 -> Write Measurement6/1
  Receive CAN Message/6 -> Write Measurement7/1
  Receive CAN Message1/6 -> Write Measurement12/1
  Receive CAN Message1/4 -> Write Measurement10/1
  Receive CAN Message1/1 -> Write Measurement8/1
  Receive CAN Message1/5 -> Write Measurement11/1
  Receive CAN Message1/2 -> Write Measurement9/1
  Receive CAN Message1/3 -> Write Measurement19/1
  Receive CAN Message2/6 -> Write Measurement15/1
  Receive CAN Message2/4 -> Write Measurement13/1
  Receive CAN Message2/1 -> Write Measurement16/1
  Receive CAN Message2/5 -> Write Measurement14/1
  Receive CAN Message2/2 -> Write Measurement17/1
  Receive CAN Message2/3 -> Write Measurement18/1

== system ECO_TestLibs/TAF_CANC/Subsystem ==
  In1 : Inport
  Logical Operator : Logic  AllPortsSameDT=off  OutDataTypeStr=boolean
  Read Calibration : CoderSF_BSW_Libs/Calibration & Measurement/Read Calibration  variable_name=TAF_CANC_flgEnRxResp_val  variable_value=1  variable_type=boolean  variable_min=[]  variable_max=[]  unitStr=""  descStr=""
      settings: AttributesFormatString=value:%<variable_value> type:%<variable_type> max:%<variable_max> Min:%<variable_min>  SourceProductName=EcoCoder Blocks
  Out1 : Outport
  wires:
  Logical Operator/1 -> Out1/1
  Read Calibration/1 -> Logical Operator/1
  In1/1 -> Logical Operator/2

== system ECO_TestLibs/TAF_CAND/Connected ==
  Read CAN Message 3 : SF_CanService_Libs/Read CAN Message  typeCAN=Connected  channel=CAN_D  mEn=off  msgInfo=TAF_CAN_new  msgIterm=CAN0x407x  msgItermStore=CAN0x407x  valid=on  stale=on  motoBit=off  setSignalName=off  defineSignalName=on  prefixSignal='rxCAND'  flgValTest=off  flgNoFixed=off  tSample=Task_L10ms  modeCode=Parameterless
  Read Fixed-Point CAN Message 3 : SF_CanService_Libs/Read Fixed-Point CAN Message   typeCAN=Connected  channel=CAN_D  mEn=off  msgInfo=TAF_CAN_new  msgIterm=CAN0x407  msgItermStore=CAN0x407  valid=on  stale=on  motoBit=off  setSignalName=on  defineSignalName=on  prefixSignal='rxCAND'  flgValTest=off  flgNoFixed=off  tSample=Task_L10ms  modeCode=Parameterless
  Subsystem3 : Subsystem
  Subsystem7 : Subsystem
  Write Measurement11 : CoderSF_BSW_Libs/Calibration & Measurement/Write Measurement  variable_name=TAF_CAN_cntCANDRx  variable_value=0  variable_type=uint32  numD=1  unitStr=""  descStr=""
      settings: AttributesFormatString=value:%<variable_value> type:%<variable_type>  SourceProductName=EcoCoder Blocks
  Write Measurement8 : CoderSF_BSW_Libs/Calibration & Measurement/Write Measurement  variable_name=TAF_CANF_cntCANDRx  variable_value=0  variable_type=uint32  numD=1  unitStr=""  descStr=""
      settings: AttributesFormatString=value:%<variable_value> type:%<variable_type>  SourceProductName=EcoCoder Blocks
  wires:
  Read CAN Message 3/1 -> Subsystem7/Enable
  Read CAN Message 3/2 -> Write Measurement11/1
  Read CAN Message 3/3 -> Subsystem7/1(In1)
  Read CAN Message 3/4 -> Subsystem7/2(In2)
  Read CAN Message 3/5 -> Subsystem7/3(In3)
  Read CAN Message 3/6 -> Subsystem7/4(In4)
  Read CAN Message 3/7 -> Subsystem7/5(In5)
  Read CAN Message 3/8 -> Subsystem7/6(In6)
  Read CAN Message 3/9 -> Subsystem7/7(In7)
  Read CAN Message 3/10 -> Subsystem7/8(In8)
  Read Fixed-Point CAN Message 3/10 -> Subsystem3/8(In8)  "rxCANDByte0"
  Read Fixed-Point CAN Message 3/9 -> Subsystem3/7(In7)  "rxCANDByte1"
  Read Fixed-Point CAN Message 3/8 -> Subsystem3/6(In6)  "rxCANDByte2"
  Read Fixed-Point CAN Message 3/7 -> Subsystem3/5(In5)  "rxCANDByte3"
  Read Fixed-Point CAN Message 3/6 -> Subsystem3/4(In4)  "rxCANDByte4"
  Read Fixed-Point CAN Message 3/5 -> Subsystem3/3(In3)  "rxCANDByte5"
  Read Fixed-Point CAN Message 3/4 -> Subsystem3/2(In2)  "rxCANDByte6"
  Read Fixed-Point CAN Message 3/3 -> Subsystem3/1(In1)  "rxCANDByte7"
  Read Fixed-Point CAN Message 3/2 -> Write Measurement8/1
  Read Fixed-Point CAN Message 3/1 -> Subsystem3/Enable

== system ECO_TestLibs/TAF_CAND/Disconnected ==
  Read CAN Message 3 : SF_CanService_Libs/Read CAN Message  typeCAN=Disconnected  channel=CAN_D  mEn=off  msgInfo=TAF_CAN_new  msgIterm=CAN0x408x  msgItermStore=CAN0x408x  valid=on  stale=on  motoBit=off  setSignalName=off  defineSignalName=on  prefixSignal='rxCAND'  flgValTest=off  flgNoFixed=off  tSample=Task_L10ms  modeCode=Parameterless
  Read Fixed-Point CAN Message 3 : SF_CanService_Libs/Read Fixed-Point CAN Message   typeCAN=Disconnected  channel=CAN_D  mEn=off  msgInfo=TAF_CAN_new  msgIterm=CAN0x408  msgItermStore=CAN0x408  valid=on  stale=on  motoBit=off  setSignalName=on  defineSignalName=on  prefixSignal='rxCAND2'  flgValTest=off  flgNoFixed=off  tSample=Task_L10ms  modeCode=Parameterless
  Receive CAN Message : CoderSF_BSW_Libs/CAN/Receive CAN Message  channel=CAN_D  txid=hex2dec('408')  extended=off  txlen=8  tasktimeIndex=Task_Inherit
      settings: SourceProductName=EcoCoder Blocks
  Receive CAN Message1 : CoderSF_BSW_Libs/CAN/Receive CAN Message  channel=CAN_D  txid=hex2dec('418')  extended=on  txlen=8  tasktimeIndex=Task_Inherit
      settings: SourceProductName=EcoCoder Blocks
  Subsystem3 : Subsystem
  Subsystem7 : Subsystem
  Write Measurement11 : CoderSF_BSW_Libs/Calibration & Measurement/Write Measurement  variable_name=TAF_CAN_cntCANDRx2  variable_value=0  variable_type=uint32  numD=1  unitStr=""  descStr=""
      settings: AttributesFormatString=value:%<variable_value> type:%<variable_type>  SourceProductName=EcoCoder Blocks
  Write Measurement8 : CoderSF_BSW_Libs/Calibration & Measurement/Write Measurement  variable_name=TAF_CANF_cntCANDRx2  variable_value=0  variable_type=uint32  numD=1  unitStr=""  descStr=""
      settings: AttributesFormatString=value:%<variable_value> type:%<variable_type>  SourceProductName=EcoCoder Blocks
  wires:
  Read Fixed-Point CAN Message 3/1 -> Subsystem3/Enable
  Read Fixed-Point CAN Message 3/2 -> Write Measurement8/1
  Read Fixed-Point CAN Message 3/3 -> Subsystem3/1(In1)  "rxCAND2Byte7"
  Read Fixed-Point CAN Message 3/4 -> Subsystem3/2(In2)  "rxCAND2Byte6"
  Read Fixed-Point CAN Message 3/5 -> Subsystem3/3(In3)  "rxCAND2Byte5"
  Read Fixed-Point CAN Message 3/6 -> Subsystem3/4(In4)  "rxCAND2Byte4"
  Read Fixed-Point CAN Message 3/7 -> Subsystem3/5(In5)  "rxCAND2Byte3"
  Read Fixed-Point CAN Message 3/8 -> Subsystem3/6(In6)  "rxCAND2Byte2"
  Read Fixed-Point CAN Message 3/9 -> Subsystem3/7(In7)  "rxCAND2Byte1"
  Read Fixed-Point CAN Message 3/10 -> Subsystem3/8(In8)  "rxCAND2Byte0"
  Read CAN Message 3/10 -> Subsystem7/8(In8)
  Read CAN Message 3/9 -> Subsystem7/7(In7)
  Read CAN Message 3/8 -> Subsystem7/6(In6)
  Read CAN Message 3/7 -> Subsystem7/5(In5)
  Read CAN Message 3/6 -> Subsystem7/4(In4)
  Read CAN Message 3/5 -> Subsystem7/3(In3)
  Read CAN Message 3/4 -> Subsystem7/2(In2)
  Read CAN Message 3/3 -> Subsystem7/1(In1)
  Read CAN Message 3/2 -> Write Measurement11/1
  Read CAN Message 3/1 -> Subsystem7/Enable
  Receive CAN Message/6 -> Read Fixed-Point CAN Message 3/6
  Receive CAN Message/4 -> Read Fixed-Point CAN Message 3/4
  Receive CAN Message/2 -> Read Fixed-Point CAN Message 3/2
  Receive CAN Message/3 -> Read Fixed-Point CAN Message 3/3
  Receive CAN Message/5 -> Read Fixed-Point CAN Message 3/5
  Receive CAN Message/1 -> Read Fixed-Point CAN Message 3/1
  Receive CAN Message1/3 -> Read CAN Message 3/3
  Receive CAN Message1/5 -> Read CAN Message 3/5
  Receive CAN Message1/4 -> Read CAN Message 3/4
  Receive CAN Message1/6 -> Read CAN Message 3/6
  Receive CAN Message1/2 -> Read CAN Message 3/2
  Receive CAN Message1/1 -> Read CAN Message 3/1
